simulink model "SimParking"  (R2017b)
settings: Solver=VariableStepAuto  StartTime=0.0  StopTime=1761  RelTol=1e-3
libraries: neural x1111
(part 3 of 60)

== system SimParking/BestNet- 10 delays -100 100 hidden neurons/Layer 2 ==
  "a{1} " : Inport  PortDimensions=100  SampleTime=1
      mask Display: e = 0.06;c1 = [120 230 180]/255;c2 = ([120 230 180]+0)/(256+128);c3 = ([120 230 180]+128)/(256+128);patch([0 1 1 0],[0 0 1 1],c1);patch([0 1 1 1-e 1-e 0+e],[0 0 1 1-e 0+e 0+e],c2);patch([0 0 1 1-e 0+e 0+e],[0 1 1 1-e 1-e 0+e],c3);plot([0 1 1 0 0],[0 0 1 1 0]);
  Delays 1 : Subsystem
      mask Display: e = 0.06;c1 = [120 150 230]/255;c2 = ([120 150 230]+0)/383;c3 = ([120 150 230]+128)/383;patch([0 1 1 0],[0 0 1 1],c1);patch([0 1 1 1-e 1-e 0+e],[0 0 1 1-e 0+e 0+e],c2);patch([0 0 1 1-e 0+e 0+e],[0 1 1 1-e 1-e 0+e],c3);plot([0 1 1 0 0],[0 0 1 1 0]);disp('0');
  "LW{2,1}" : Subsystem
      mask Display: e = 0.06;c1 = [120 150 230]/255;c2 = ([120 150 230]+0)/383;c3 = ([120 150 230]+128)/383;patch([0 1 1 0],[0 0 1 1],c1);patch([0 1 1 1-e 1-e 0+e],[0 0 1 1-e 0+e 0+e],c2);patch([0 0 1 1-e 0+e 0+e],[0 1 1 1-e 1-e 0+e],c3);plot([0 1 1 0 0],[0 0 1 1 0]);disp('W');
  "b{2}" : Constant  Value=[-1.5233467696368359067804476580931805074214935302734375;-1.4415804453285188113653703112504445016384124755859375;1.4687499329954964988331767017371021211147308349609375;1.378535301430398707367430688464082777500152587890625;1.4334155218379340812617783740279264748096466064453125;-1.3690887831616393999212277776678092777729034423828125;-1.304160375402110272347044883645139634609222412109375;1.29600772472264846868483800790272653102874755859375;1.2498985632110517496329293862800113856792449951171875;1.2638509294992459341955282070557586848735809326171875;1.208129855846170830346864022430963814258575439453125;1.1824187437823148183468902061576955020427703857421875;1.160993267964341324471888583502732217311859130859375;1.10675966022170069180674545350484549999237060546875;-1.105033867711343820161573603400029242038726806640625;1.032881951698968681085943899233825504779815673828125;-0.98852583000171645455367297472548671066761016845703125;-1.003489835974161525911085846018977463245391845703125;-0.94450071591520201597091954681673087179660797119140625;-0.96655837310848158328013823847868479788303375244140625;-0.8538722720434481772144863498397171497344970703125;0.8426292105943014032476412467076443135738372802734375;-0.8802935092119688054168591406778432428836822509765625;-0.81787353156131759046587603734224103391170501708984375;-0.7137736873323863306950443075038492679595947265625;-0.7368245035904037454344006619066931307315826416015625;-0.66775958311495842156801927558262832462787628173828125;-0.57961887312592608179073749852250330150127410888671875;0.67555184756865627182520483984262682497501373291015625;0.68969451052878183450189908398897387087345123291015625;0.61762410004044998590444492947426624596118927001953125;0.6022014857071804616595045445137657225131988525390625;-0.526192511812102026169668533839285373687744140625;0.51561667677955635991082772306981496512889862060546875;-0.414470085354920747544582582122529856860637664794921875;-0.43640562865662513303277592058293521404266357421875;-0.4769010705651643977631692905561067163944244384765625;0.30156500972384758796351889031939208507537841796875;0.380377257082855357861461698121274821460247039794921875;-0.256097557968687272733632198651321232318878173828125;0.25819514267073084834436258461209945380687713623046875;0.239800622449258538093630477305850945413112640380859375;0.238207291683244115620965430935029871761798858642578125;-0.2465816261413751597775245727461879141628742218017578125;0.2765787596096604961104503672686405479907989501953125;0.08005536680915757707932556286323233507573604583740234375;-0.1529351096854706659744493890684680081903934478759765625;0.11905624484543265995117877764641889370977878570556640625;0.09813681425791646872891504926883499138057231903076171875;-0.0679352414639936286189225711495964787900447845458984375;-0.06834830466920095715099847666351706720888614654541015625;-0.156043028201395816978447328438051044940948486328125;0.0237726502873336666132875194534790352918207645416259765625;-0.034534939705202348514401222701053484342992305755615234375;-0.042901038724158180315271238214336335659027099609375;0.1717782700492356540156180244593997485935688018798828125;0.1147508327533348360116605135772260837256908416748046875;-0.254165471349188598626511748079792596399784088134765625;0.2069296799639553097183153340665739960968494415283203125;-0.29569483453317657595249556834460236132144927978515625;0.388897541037930560836599624963128007948398590087890625;-0.373484441161281266463589645354659296572208404541015625;-0.363064211852830276416881361001287586987018585205078125;-0.40194412444326232947133803463657386600971221923828125;0.52257111750173967923416284975246526300907135009765625;-0.4052040280159545648785979210515506565570831298828125;0.4311907495262088385601373374811373651027679443359375;0.623613308142939803957460753736086189746856689453125;-0.485832292806824661557385525156860239803791046142578125;-0.66397809913526162350905224229791201651096343994140625;-0.672562449456481470377866571652702987194061279296875 ...(+1576 chars)]
      mask Display: e = 0.06;c1 = [120 150 230]/255;c2 = ([120 150 230]+0)/383;c3 = ([120 150 230]+128)/383;patch([0 1 1 0],[0 0 1 1],c1);patch([0 1 1 1-e 1-e 0+e],[0 0 1 1-e 0+e 0+e],c2);patch([0 0 1 1-e 0+e 0+e],[0 1 1 1-e 1-e 0+e],c3);plot([0 1 1 0 0],[0 0 1 1 0]);disp('b');
  netsum : Sum  Inputs=2  SaturateOnIntegerOverflow=on  InputSameDT=on  OutDataTypeStr=Inherit: Same as first input
      mask Display: e = 0.06;c1 = [120 150 230]/255;c2 = ([120 150 230]+0)/383;c3 = ([120 150 230]+128)/383;patch([0 1 1 0],[0 0 1 1],c1);patch([0 1 1 1-e 1-e 0+e],[0 0 1 1-e 0+e 0+e],c2);patch([0 0 1 1-e 0+e 0+e],[0 1 1 1-e 1-e 0+e],c3);plot([0 1 1 0 0],[0 0 1 1 0]);disp('+');
  tansig : neural/Transfer Functions/tansig
  "a{2}" : Outport  InitialOutput=[0;0;0;0;0;0;0;0;0;0;0;0;0;0;0;0;0;0;0;0;0;0;0;0;0;0;0;0;0;0;0;0;0;0;0;0;0;0;0;0;0;0;0;0;0;0;0;0;0;0;0;0;0;0;0;0;0;0;0;0;0;0;0;0;0;0;0;0;0;0;0;0;0;0;0;0;0;0;0;0;0;0;0;0;0;0;0;0;0;0;0;0;0;0;0;0;0;0;0;0]
      mask Display: e = 0.06;c1 = [120 230 180]/255;c2 = ([120 230 180]+0)/(256+128);c3 = ([120 230 180]+128)/(256+128);patch([0 1 1 0],[0 0 1 1],c1);patch([0 1 1 1-e 1-e 0+e],[0 0 1 1-e 0+e 0+e],c2);patch([0 0 1 1-e 0+e 0+e],[0 1 1 1-e 1-e 0+e],c3);plot([0 1 1 0 0],[0 0 1 1 0]);
  wires:
  "a{1} "/1 -> Delays 1/1("p{2}")
  Delays 1/1("pd{2,1}") -> "LW{2,1}"/1("ad{2,1}")
  "LW{2,1}"/1("lz{2,1}") -> netsum/1
  "b{2}"/1 -> netsum/2
  netsum/1 -> tansig/1
  tansig/1 -> "a{2}"/1

== system SimParking/BestNet- 10 delays -100 100 hidden neurons/Layer 3 ==
  "a{2} " : Inport  PortDimensions=100  SampleTime=1
      mask Display: e = 0.06;c1 = [120 230 180]/255;c2 = ([120 230 180]+0)/(256+128);c3 = ([120 230 180]+128)/(256+128);patch([0 1 1 0],[0 0 1 1],c1);patch([0 1 1 1-e 1-e 0+e],[0 0 1 1-e 0+e 0+e],c2);patch([0 0 1 1-e 0+e 0+e],[0 1 1 1-e 1-e 0+e],c3);plot([0 1 1 0 0],[0 0 1 1 0]);
  Delays 1 : Subsystem
      mask Display: e = 0.06;c1 = [120 150 230]/255;c2 = ([120 150 230]+0)/383;c3 = ([120 150 230]+128)/383;patch([0 1 1 0],[0 0 1 1],c1);patch([0 1 1 1-e 1-e 0+e],[0 0 1 1-e 0+e 0+e],c2);patch([0 0 1 1-e 0+e 0+e],[0 1 1 1-e 1-e 0+e],c3);plot([0 1 1 0 0],[0 0 1 1 0]);disp('0');
  "LW{3,2}" : Subsystem
      mask Display: e = 0.06;c1 = [120 150 230]/255;c2 = ([120 150 230]+0)/383;c3 = ([120 150 230]+128)/383;patch([0 1 1 0],[0 0 1 1],c1);patch([0 1 1 1-e 1-e 0+e],[0 0 1 1-e 0+e 0+e],c2);patch([0 0 1 1-e 0+e 0+e],[0 1 1 1-e 1-e 0+e],c3);plot([0 1 1 0 0],[0 0 1 1 0]);disp('W');
  "b{3}" : Constant  Value=[-0.264399040939169382991025258888839744031429290771484375;-0.2280200632373896307836247387967887334525585174560546875;0.1500776635383979928928255276332492940127849578857421875]
      mask Display: e = 0.06;c1 = [120 150 230]/255;c2 = ([120 150 230]+0)/383;c3 = ([120 150 230]+128)/383;patch([0 1 1 0],[0 0 1 1],c1);patch([0 1 1 1-e 1-e 0+e],[0 0 1 1-e 0+e 0+e],c2);patch([0 0 1 1-e 0+e 0+e],[0 1 1 1-e 1-e 0+e],c3);plot([0 1 1 0 0],[0 0 1 1 0]);disp('b');
  netsum : Sum  Inputs=2  SaturateOnIntegerOverflow=on  InputSameDT=on  OutDataTypeStr=Inherit: Same as first input
      mask Display: e = 0.06;c1 = [120 150 230]/255;c2 = ([120 150 230]+0)/383;c3 = ([120 150 230]+128)/383;patch([0 1 1 0],[0 0 1 1],c1);patch([0 1 1 1-e 1-e 0+e],[0 0 1 1-e 0+e 0+e],c2);patch([0 0 1 1-e 0+e 0+e],[0 1 1 1-e 1-e 0+e],c3);plot([0 1 1 0 0],[0 0 1 1 0]);disp('+');
  purelin : neural/Transfer Functions/purelin
  "a{3}" : Outport  InitialOutput=[0;0;0]
      mask Display: e = 0.06;c1 = [120 230 180]/255;c2 = ([120 230 180]+0)/(256+128);c3 = ([120 230 180]+128)/(256+128);patch([0 1 1 0],[0 0 1 1],c1);patch([0 1 1 1-e 1-e 0+e],[0 0 1 1-e 0+e 0+e],c2);patch([0 0 1 1-e 0+e 0+e],[0 1 1 1-e 1-e 0+e],c3);plot([0 1 1 0 0],[0 0 1 1 0]);
  wires:
  "a{2} "/1 -> Delays 1/1("p{3}")
  Delays 1/1("pd{3,2}") -> "LW{3,2}"/1("ad{3,2}")
  "LW{3,2}"/1("lz{3,2}") -> netsum/1
  "b{3}"/1 -> netsum/2
  netsum/1 -> purelin/1
  purelin/1 -> "a{3}"/1

== system SimParking/BestNet- 10 delays -100 100 hidden neurons/Process Input 1 ==
  x : Inport  PortDimensions=9  SampleTime=1
      mask Display: e = 0.06;c1 = [120 230 180]/255;c2 = ([120 230 180]+0)/(256+128);c3 = ([120 230 180]+128)/(256+128);patch([0 1 1 0],[0 0 1 1],c1);patch([0 1 1 1-e 1-e 0+e],[0 0 1 1-e 0+e 0+e],c2);patch([0 0 1 1-e 0+e 0+e],[0 1 1 1-e 1-e 0+e],c3);plot([0 1 1 0 0],[0 0 1 1 0]);
  mapminmax : neural/Processing Functions/mapminmax  xmin=[0;-0.00100000000000000002081668171172;-0.927000000000000046185277824407;-0.0367373000000000005105249556436;0;0;0;0;0]  xmax=[1;4.75300000000000011368683772162;0;1.1136800000000000032684965845;2.19799999999999995381472217559;1;1;1;1]  ymin=-1  ymax=1
  p : Outport  PortDimensions=9  SampleTime=1
      mask Display: e = 0.06;c1 = [120 230 180]/255;c2 = ([120 230 180]+0)/(256+128);c3 = ([120 230 180]+128)/(256+128);patch([0 1 1 0],[0 0 1 1],c1);patch([0 1 1 1-e 1-e 0+e],[0 0 1 1-e 0+e 0+e],c2);patch([0 0 1 1-e 0+e 0+e],[0 1 1 1-e 1-e 0+e],c3);plot([0 1 1 0 0],[0 0 1 1 0]);
  wires:
  x/1 -> mapminmax/1
  mapminmax/1 -> p/1

== system SimParking/BestNet- 10 delays -100 100 hidden neurons/Process Output 1 ==
  a : Inport  PortDimensions=3  SampleTime=1
      mask Display: e = 0.06;c1 = [120 230 180]/255;c2 = ([120 230 180]+0)/(256+128);c3 = ([120 230 180]+128)/(256+128);patch([0 1 1 0],[0 0 1 1],c1);patch([0 1 1 1-e 1-e 0+e],[0 0 1 1-e 0+e 0+e],c2);patch([0 0 1 1-e 0+e 0+e],[0 1 1 1-e 1-e 0+e],c3);plot([0 1 1 0 0],[0 0 1 1 0]);
  mapminmax_reverse : neural/Processing Functions/mapminmax_reverse  xmin=[-0.142810999999999993503863038313;-0.169776000000000010237144465464;0]  xmax=[0.231192000000000008608225243734;0.179999999999999993338661852249;1]  ymin=-1  ymax=1
  y : Outport  PortDimensions=3  SampleTime=1
      mask Display: e = 0.06;c1 = [120 230 180]/255;c2 = ([120 230 180]+0)/(256+128);c3 = ([120 230 180]+128)/(256+128);patch([0 1 1 0],[0 0 1 1],c1);patch([0 1 1 1-e 1-e 0+e],[0 0 1 1-e 0+e 0+e],c2);patch([0 0 1 1-e 0+e 0+e],[0 1 1 1-e 1-e 0+e],c3);plot([0 1 1 0 0],[0 0 1 1 0]);
  wires:
  a/1 -> mapminmax_reverse/1
  mapminmax_reverse/1 -> y/1

== system SimParking/BestNet- 10 delays -100 100 hidden neurons1/Layer 1 ==
  "p{1}" : Inport  PortDimensions=9  SampleTime=1
      mask Display: e = 0.06;c1 = [120 230 180]/255;c2 = ([120 230 180]+0)/(256+128);c3 = ([120 230 180]+128)/(256+128);patch([0 1 1 0],[0 0 1 1],c1);patch([0 1 1 1-e 1-e 0+e],[0 0 1 1-e 0+e 0+e],c2);patch([0 0 1 1-e 0+e 0+e],[0 1 1 1-e 1-e 0+e],c3);plot([0 1 1 0 0],[0 0 1 1 0]);
  Delays 1 : Subsystem
      mask Display: e = 0.06;c1 = [120 150 230]/255;c2 = ([120 150 230]+0)/383;c3 = ([120 150 230]+128)/383;patch([0 1 1 0],[0 0 1 1],c1);patch([0 1 1 1-e 1-e 0+e],[0 0 1 1-e 0+e 0+e],c2);patch([0 0 1 1-e 0+e 0+e],[0 1 1 1-e 1-e 0+e],c3);plot([0 1 1 0 0],[0 0 1 1 0]);disp('1-10');
  "IW{1,1}" : Subsystem
      mask Display: e = 0.06;c1 = [120 150 230]/255;c2 = ([120 150 230]+0)/383;c3 = ([120 150 230]+128)/383;patch([0 1 1 0],[0 0 1 1],c1);patch([0 1 1 1-e 1-e 0+e],[0 0 1 1-e 0+e 0+e],c2);patch([0 0 1 1-e 0+e 0+e],[0 1 1 1-e 1-e 0+e],c3);plot([0 1 1 0 0],[0 0 1 1 0]);disp('W');
  "b{1}" : Constant  Value=[-1.5245225286757662086500886289286427199840545654296875;1.6058316686755433888578181722550652921199798583984375;1.517403103952690290867622024961747229099273681640625;-1.386904812575269207997052944847382605075836181640625;-1.3545623995403683892391200060956180095672607421875;1.470857444827213367233298413339070975780487060546875;-1.2857387543680351971175923608825542032718658447265625;-1.359082929289666452632445725612342357635498046875;-1.3064762119514614635562566036242060363292694091796875;-1.22721098835727193687716862768866121768951416015625;1.2308531077143507470594840924604795873165130615234375;1.336790839668508201754093533963896334171295166015625;1.11248789445838536238397864508442580699920654296875;1.161779163995248609353438951075077056884765625;-1.11085814127999693567971917218528687953948974609375;-1.16588845394895290752401706413365900516510009765625;0.978431286318926396461392869241535663604736328125;-1.0267597507064201156623539645806886255741119384765625;-1.0466534182444442446779930833145044744014739990234375;1.05098808141578725638964897370897233486175537109375;0.93621859385301731126816093819797970354557037353515625;-1.000511208787383310436780448071658611297607421875;-0.90766483038739564914720858723740093410015106201171875;-0.84546048837210940885000809430493973195552825927734375;0.84876630264789287849680476938374340534210205078125;-0.80185690636105755313423060215427540242671966552734375;-0.5148210028828319462235185710596852004528045654296875;-0.65524102483332169466478944741538725793361663818359375;0.715828663178128099531249972642399370670318603515625;0.547477588095126588285666002775542438030242919921875;0.6337090972519561216103056722204200923442840576171875;0.61282296794795898531305056167184375226497650146484375;-0.62963945517072217317178228768170811235904693603515625;-0.5600633886452470733274822123348712921142578125;-0.5142547132588661806806840104400180280208587646484375;0.36622414618450871426347248416277579963207244873046875;0.435171860018647882473175059203640557825565338134765625;-0.3973775967826436161800529589527286589145660400390625;-0.412985049052973895999940623369184322655200958251953125;-0.456498738819200500227424299737322144210338592529296875;-0.368563532068655719253769120768993161618709564208984375;-0.1451264394857011696959858682021149434149265289306640625;0.2374280696468461793191551123527460731565952301025390625;0.169516230719349125788397714131860993802547454833984375;-0.01207776799942027710910164017832357785664498805999755859375;0.07982326989852468746011737721346435137093067169189453125;0.18978690166193568078512043939554132521152496337890625;0.1312090183858221903445695488699129782617092132568359375;-0.13599776027038201764440827901125885546207427978515625;0.0259802672083776220457451699985540471971035003662109375;0.09588393978311908483203040987064014188945293426513671875;-0.000439077264281844520908693052518856347887776792049407958984375;0.10623277174090879626522365697383065707981586456298828125;-0.1382214176826130069830611546422005631029605865478515625;0.128992117787592286415332409887923859059810638427734375;-0.0820858742952841613504944007218000479042530059814453125;-0.1798165459899483398231723185745067894458770751953125;-0.386315691932279381415327179638552479445934295654296875;0.18505331061093144295881529615144245326519012451171875;-0.276070952220042686864331926699378527700901031494140625;0.1470903025261399432732645209398469887673854827880859375;0.355437619732055509746970756168593652546405792236328125;-0.33831043495201262860661017839447595179080963134765625;-0.507272391830840607696018196293152868747711181640625;0.459441289358410720478076427752966992557048797607421875;0.424515668838529147688376497171702794730663299560546875;0.63498576332306655434223330303211696445941925048828125;0.487893153924136402377342847103136591613292694091796875;0.69410429992965394507820064973202534019947052001953125;0.751872227891053679371680118492804467678070068359375;-0.82872934292105782105863909237086772918701171875 ...(+1580 chars)]
      mask Display: e = 0.06;c1 = [120 150 230]/255;c2 = ([120 150 230]+0)/383;c3 = ([120 150 230]+128)/383;patch([0 1 1 0],[0 0 1 1],c1);patch([0 1 1 1-e 1-e 0+e],[0 0 1 1-e 0+e 0+e],c2);patch([0 0 1 1-e 0+e 0+e],[0 1 1 1-e 1-e 0+e],c3);plot([0 1 1 0 0],[0 0 1 1 0]);disp('b');
  netsum : Sum  Inputs=2  SaturateOnIntegerOverflow=on  InputSameDT=on  OutDataTypeStr=Inherit: Same as first input
      mask Display: e = 0.06;c1 = [120 150 230]/255;c2 = ([120 150 230]+0)/383;c3 = ([120 150 230]+128)/383;patch([0 1 1 0],[0 0 1 1],c1);patch([0 1 1 1-e 1-e 0+e],[0 0 1 1-e 0+e 0+e],c2);patch([0 0 1 1-e 0+e 0+e],[0 1 1 1-e 1-e 0+e],c3);plot([0 1 1 0 0],[0 0 1 1 0]);disp('+');
  tansig : neural/Transfer Functions/tansig
  "a{1}" : Outport  InitialOutput=[0;0;0;0;0;0;0;0;0;0;0;0;0;0;0;0;0;0;0;0;0;0;0;0;0;0;0;0;0;0;0;0;0;0;0;0;0;0;0;0;0;0;0;0;0;0;0;0;0;0;0;0;0;0;0;0;0;0;0;0;0;0;0;0;0;0;0;0;0;0;0;0;0;0;0;0;0;0;0;0;0;0;0;0;0;0;0;0;0;0;0;0;0;0;0;0;0;0;0;0]
      mask Display: e = 0.06;c1 = [120 230 180]/255;c2 = ([120 230 180]+0)/(256+128);c3 = ([120 230 180]+128)/(256+128);patch([0 1 1 0],[0 0 1 1],c1);patch([0 1 1 1-e 1-e 0+e],[0 0 1 1-e 0+e 0+e],c2);patch([0 0 1 1-e 0+e 0+e],[0 1 1 1-e 1-e 0+e],c3);plot([0 1 1 0 0],[0 0 1 1 0]);
  wires:
  "p{1}"/1 -> Delays 1/1("p{1}")
  Delays 1/1("pd{1,1}") -> "IW{1,1}"/1("pd{1,1}")
  "IW{1,1}"/1("iz{1,1}") -> netsum/1
  "b{1}"/1 -> netsum/2
  netsum/1 -> tansig/1
  tansig/1 -> "a{1}"/1

== system SimParking/BestNet- 10 delays -100 100 hidden neurons1/Layer 2 ==
  "a{1} " : Inport  PortDimensions=100  SampleTime=1
      mask Display: e = 0.06;c1 = [120 230 180]/255;c2 = ([120 230 180]+0)/(256+128);c3 = ([120 230 180]+128)/(256+128);patch([0 1 1 0],[0 0 1 1],c1);patch([0 1 1 1-e 1-e 0+e],[0 0 1 1-e 0+e 0+e],c2);patch([0 0 1 1-e 0+e 0+e],[0 1 1 1-e 1-e 0+e],c3);plot([0 1 1 0 0],[0 0 1 1 0]);
  Delays 1 : Subsystem
      mask Display: e = 0.06;c1 = [120 150 230]/255;c2 = ([120 150 230]+0)/383;c3 = ([120 150 230]+128)/383;patch([0 1 1 0],[0 0 1 1],c1);patch([0 1 1 1-e 1-e 0+e],[0 0 1 1-e 0+e 0+e],c2);patch([0 0 1 1-e 0+e 0+e],[0 1 1 1-e 1-e 0+e],c3);plot([0 1 1 0 0],[0 0 1 1 0]);disp('0');
  "LW{2,1}" : Subsystem
      mask Display: e = 0.06;c1 = [120 150 230]/255;c2 = ([120 150 230]+0)/383;c3 = ([120 150 230]+128)/383;patch([0 1 1 0],[0 0 1 1],c1);patch([0 1 1 1-e 1-e 0+e],[0 0 1 1-e 0+e 0+e],c2);patch([0 0 1 1-e 0+e 0+e],[0 1 1 1-e 1-e 0+e],c3);plot([0 1 1 0 0],[0 0 1 1 0]);disp('W');
  "b{2}" : Constant  Value=[-1.5233467696368359067804476580931805074214935302734375;-1.4415804453285188113653703112504445016384124755859375;1.4687499329954964988331767017371021211147308349609375;1.378535301430398707367430688464082777500152587890625;1.4334155218379340812617783740279264748096466064453125;-1.3690887831616393999212277776678092777729034423828125;-1.304160375402110272347044883645139634609222412109375;1.29600772472264846868483800790272653102874755859375;1.2498985632110517496329293862800113856792449951171875;1.2638509294992459341955282070557586848735809326171875;1.208129855846170830346864022430963814258575439453125;1.1824187437823148183468902061576955020427703857421875;1.160993267964341324471888583502732217311859130859375;1.10675966022170069180674545350484549999237060546875;-1.105033867711343820161573603400029242038726806640625;1.032881951698968681085943899233825504779815673828125;-0.98852583000171645455367297472548671066761016845703125;-1.003489835974161525911085846018977463245391845703125;-0.94450071591520201597091954681673087179660797119140625;-0.96655837310848158328013823847868479788303375244140625;-0.8538722720434481772144863498397171497344970703125;0.8426292105943014032476412467076443135738372802734375;-0.8802935092119688054168591406778432428836822509765625;-0.81787353156131759046587603734224103391170501708984375;-0.7137736873323863306950443075038492679595947265625;-0.7368245035904037454344006619066931307315826416015625;-0.66775958311495842156801927558262832462787628173828125;-0.57961887312592608179073749852250330150127410888671875;0.67555184756865627182520483984262682497501373291015625;0.68969451052878183450189908398897387087345123291015625;0.61762410004044998590444492947426624596118927001953125;0.6022014857071804616595045445137657225131988525390625;-0.526192511812102026169668533839285373687744140625;0.51561667677955635991082772306981496512889862060546875;-0.414470085354920747544582582122529856860637664794921875;-0.43640562865662513303277592058293521404266357421875;-0.4769010705651643977631692905561067163944244384765625;0.30156500972384758796351889031939208507537841796875;0.380377257082855357861461698121274821460247039794921875;-0.256097557968687272733632198651321232318878173828125;0.25819514267073084834436258461209945380687713623046875;0.239800622449258538093630477305850945413112640380859375;0.238207291683244115620965430935029871761798858642578125;-0.2465816261413751597775245727461879141628742218017578125;0.2765787596096604961104503672686405479907989501953125;0.08005536680915757707932556286323233507573604583740234375;-0.1529351096854706659744493890684680081903934478759765625;0.11905624484543265995117877764641889370977878570556640625;0.09813681425791646872891504926883499138057231903076171875;-0.0679352414639936286189225711495964787900447845458984375;-0.06834830466920095715099847666351706720888614654541015625;-0.156043028201395816978447328438051044940948486328125;0.0237726502873336666132875194534790352918207645416259765625;-0.034534939705202348514401222701053484342992305755615234375;-0.042901038724158180315271238214336335659027099609375;0.1717782700492356540156180244593997485935688018798828125;0.1147508327533348360116605135772260837256908416748046875;-0.254165471349188598626511748079792596399784088134765625;0.2069296799639553097183153340665739960968494415283203125;-0.29569483453317657595249556834460236132144927978515625;0.388897541037930560836599624963128007948398590087890625;-0.373484441161281266463589645354659296572208404541015625;-0.363064211852830276416881361001287586987018585205078125;-0.40194412444326232947133803463657386600971221923828125;0.52257111750173967923416284975246526300907135009765625;-0.4052040280159545648785979210515506565570831298828125;0.4311907495262088385601373374811373651027679443359375;0.623613308142939803957460753736086189746856689453125;-0.485832292806824661557385525156860239803791046142578125;-0.66397809913526162350905224229791201651096343994140625;-0.672562449456481470377866571652702987194061279296875 ...(+1576 chars)]
      mask Display: e = 0.06;c1 = [120 150 230]/255;c2 = ([120 150 230]+0)/383;c3 = ([120 150 230]+128)/383;patch([0 1 1 0],[0 0 1 1],c1);patch([0 1 1 1-e 1-e 0+e],[0 0 1 1-e 0+e 0+e],c2);patch([0 0 1 1-e 0+e 0+e],[0 1 1 1-e 1-e 0+e],c3);plot([0 1 1 0 0],[0 0 1 1 0]);disp('b');
  netsum : Sum  Inputs=2  SaturateOnIntegerOverflow=on  InputSameDT=on  OutDataTypeStr=Inherit: Same as first input
      mask Display: e = 0.06;c1 = [120 150 230]/255;c2 = ([120 150 230]+0)/383;c3 = ([120 150 230]+128)/383;patch([0 1 1 0],[0 0 1 1],c1);patch([0 1 1 1-e 1-e 0+e],[0 0 1 1-e 0+e 0+e],c2);patch([0 0 1 1-e 0+e 0+e],[0 1 1 1-e 1-e 0+e],c3);plot([0 1 1 0 0],[0 0 1 1 0]);disp('+');
  tansig : neural/Transfer Functions/tansig
  "a{2}" : Outport  InitialOutput=[0;0;0;0;0;0;0;0;0;0;0;0;0;0;0;0;0;0;0;0;0;0;0;0;0;0;0;0;0;0;0;0;0;0;0;0;0;0;0;0;0;0;0;0;0;0;0;0;0;0;0;0;0;0;0;0;0;0;0;0;0;0;0;0;0;0;0;0;0;0;0;0;0;0;0;0;0;0;0;0;0;0;0;0;0;0;0;0;0;0;0;0;0;0;0;0;0;0;0;0]
      mask Display: e = 0.06;c1 = [120 230 180]/255;c2 = ([120 230 180]+0)/(256+128);c3 = ([120 230 180]+128)/(256+128);patch([0 1 1 0],[0 0 1 1],c1);patch([0 1 1 1-e 1-e 0+e],[0 0 1 1-e 0+e 0+e],c2);patch([0 0 1 1-e 0+e 0+e],[0 1 1 1-e 1-e 0+e],c3);plot([0 1 1 0 0],[0 0 1 1 0]);
  wires:
  "a{1} "/1 -> Delays 1/1("p{2}")
  Delays 1/1("pd{2,1}") -> "LW{2,1}"/1("ad{2,1}")
  "LW{2,1}"/1("lz{2,1}") -> netsum/1
  "b{2}"/1 -> netsum/2
  netsum/1 -> tansig/1
  tansig/1 -> "a{2}"/1

== system SimParking/BestNet- 10 delays -100 100 hidden neurons1/Layer 3 ==
  "a{2} " : Inport  PortDimensions=100  SampleTime=1
      mask Display: e = 0.06;c1 = [120 230 180]/255;c2 = ([120 230 180]+0)/(256+128);c3 = ([120 230 180]+128)/(256+128);patch([0 1 1 0],[0 0 1 1],c1);patch([0 1 1 1-e 1-e 0+e],[0 0 1 1-e 0+e 0+e],c2);patch([0 0 1 1-e 0+e 0+e],[0 1 1 1-e 1-e 0+e],c3);plot([0 1 1 0 0],[0 0 1 1 0]);
  Delays 1 : Subsystem
      mask Display: e = 0.06;c1 = [120 150 230]/255;c2 = ([120 150 230]+0)/383;c3 = ([120 150 230]+128)/383;patch([0 1 1 0],[0 0 1 1],c1);patch([0 1 1 1-e 1-e 0+e],[0 0 1 1-e 0+e 0+e],c2);patch([0 0 1 1-e 0+e 0+e],[0 1 1 1-e 1-e 0+e],c3);plot([0 1 1 0 0],[0 0 1 1 0]);disp('0');
  "LW{3,2}" : Subsystem
      mask Display: e = 0.06;c1 = [120 150 230]/255;c2 = ([120 150 230]+0)/383;c3 = ([120 150 230]+128)/383;patch([0 1 1 0],[0 0 1 1],c1);patch([0 1 1 1-e 1-e 0+e],[0 0 1 1-e 0+e 0+e],c2);patch([0 0 1 1-e 0+e 0+e],[0 1 1 1-e 1-e 0+e],c3);plot([0 1 1 0 0],[0 0 1 1 0]);disp('W');
  "b{3}" : Constant  Value=[-0.264399040939169382991025258888839744031429290771484375;-0.2280200632373896307836247387967887334525585174560546875;0.1500776635383979928928255276332492940127849578857421875]
      mask Display: e = 0.06;c1 = [120 150 230]/255;c2 = ([120 150 230]+0)/383;c3 = ([120 150 230]+128)/383;patch([0 1 1 0],[0 0 1 1],c1);patch([0 1 1 1-e 1-e 0+e],[0 0 1 1-e 0+e 0+e],c2);patch([0 0 1 1-e 0+e 0+e],[0 1 1 1-e 1-e 0+e],c3);plot([0 1 1 0 0],[0 0 1 1 0]);disp('b');
  netsum : Sum  Inputs=2  SaturateOnIntegerOverflow=on  InputSameDT=on  OutDataTypeStr=Inherit: Same as first input
      mask Display: e = 0.06;c1 = [120 150 230]/255;c2 = ([120 150 230]+0)/383;c3 = ([120 150 230]+128)/383;patch([0 1 1 0],[0 0 1 1],c1);patch([0 1 1 1-e 1-e 0+e],[0 0 1 1-e 0+e 0+e],c2);patch([0 0 1 1-e 0+e 0+e],[0 1 1 1-e 1-e 0+e],c3);plot([0 1 1 0 0],[0 0 1 1 0]);disp('+');
  purelin : neural/Transfer Functions/purelin
  "a{3}" : Outport  InitialOutput=[0;0;0]
      mask Display: e = 0.06;c1 = [120 230 180]/255;c2 = ([120 230 180]+0)/(256+128);c3 = ([120 230 180]+128)/(256+128);patch([0 1 1 0],[0 0 1 1],c1);patch([0 1 1 1-e 1-e 0+e],[0 0 1 1-e 0+e 0+e],c2);patch([0 0 1 1-e 0+e 0+e],[0 1 1 1-e 1-e 0+e],c3);plot([0 1 1 0 0],[0 0 1 1 0]);
  wires:
  "a{2} "/1 -> Delays 1/1("p{3}")
  Delays 1/1("pd{3,2}") -> "LW{3,2}"/1("ad{3,2}")
  "LW{3,2}"/1("lz{3,2}") -> netsum/1
  "b{3}"/1 -> netsum/2
  netsum/1 -> purelin/1
  purelin/1 -> "a{3}"/1

== system SimParking/BestNet- 10 delays -100 100 hidden neurons1/Process Input 1 ==
  x : Inport  PortDimensions=9  SampleTime=1
      mask Display: e = 0.06;c1 = [120 230 180]/255;c2 = ([120 230 180]+0)/(256+128);c3 = ([120 230 180]+128)/(256+128);patch([0 1 1 0],[0 0 1 1],c1);patch([0 1 1 1-e 1-e 0+e],[0 0 1 1-e 0+e 0+e],c2);patch([0 0 1 1-e 0+e 0+e],[0 1 1 1-e 1-e 0+e],c3);plot([0 1 1 0 0],[0 0 1 1 0]);
  mapminmax : neural/Processing Functions/mapminmax  xmin=[0;-0.00100000000000000002081668171172;-0.927000000000000046185277824407;-0.0367373000000000005105249556436;0;0;0;0;0]  xmax=[1;4.75300000000000011368683772162;0;1.1136800000000000032684965845;2.19799999999999995381472217559;1;1;1;1]  ymin=-1  ymax=1
  p : Outport  PortDimensions=9  SampleTime=1
      mask Display: e = 0.06;c1 = [120 230 180]/255;c2 = ([120 230 180]+0)/(256+128);c3 = ([120 230 180]+128)/(256+128);patch([0 1 1 0],[0 0 1 1],c1);patch([0 1 1 1-e 1-e 0+e],[0 0 1 1-e 0+e 0+e],c2);patch([0 0 1 1-e 0+e 0+e],[0 1 1 1-e 1-e 0+e],c3);plot([0 1 1 0 0],[0 0 1 1 0]);
  wires:
  x/1 -> mapminmax/1
  mapminmax/1 -> p/1

== system SimParking/BestNet- 10 delays -100 100 hidden neurons1/Process Output 1 ==
  a : Inport  PortDimensions=3  SampleTime=1
      mask Display: e = 0.06;c1 = [120 230 180]/255;c2 = ([120 230 180]+0)/(256+128);c3 = ([120 230 180]+128)/(256+128);patch([0 1 1 0],[0 0 1 1],c1);patch([0 1 1 1-e 1-e 0+e],[0 0 1 1-e 0+e 0+e],c2);patch([0 0 1 1-e 0+e 0+e],[0 1 1 1-e 1-e 0+e],c3);plot([0 1 1 0 0],[0 0 1 1 0]);
  mapminmax_reverse : neural/Processing Functions/mapminmax_reverse  xmin=[-0.142810999999999993503863038313;-0.169776000000000010237144465464;0]  xmax=[0.231192000000000008608225243734;0.179999999999999993338661852249;1]  ymin=-1  ymax=1
  y : Outport  PortDimensions=3  SampleTime=1
      mask Display: e = 0.06;c1 = [120 230 180]/255;c2 = ([120 230 180]+0)/(256+128);c3 = ([120 230 180]+128)/(256+128);patch([0 1 1 0],[0 0 1 1],c1);patch([0 1 1 1-e 1-e 0+e],[0 0 1 1-e 0+e 0+e],c2);patch([0 0 1 1-e 0+e 0+e],[0 1 1 1-e 1-e 0+e],c3);plot([0 1 1 0 0],[0 0 1 1 0]);
  wires:
  a/1 -> mapminmax_reverse/1
  mapminmax_reverse/1 -> y/1

== system SimParking/NARX Neural Network/Layer 1 ==
  "p{1}" : Inport  PortDimensions=9  SampleTime=1
      mask Display: e = 0.06;c1 = [120 230 180]/255;c2 = ([120 230 180]+0)/(256+128);c3 = ([120 230 180]+128)/(256+128);patch([0 1 1 0],[0 0 1 1],c1);patch([0 1 1 1-e 1-e 0+e],[0 0 1 1-e 0+e 0+e],c2);patch([0 0 1 1-e 0+e 0+e],[0 1 1 1-e 1-e 0+e],c3);plot([0 1 1 0 0],[0 0 1 1 0]);
  "p{2}" : Inport  Port=2  PortDimensions=3  SampleTime=1
      mask Display: e = 0.06;c1 = [120 230 180]/255;c2 = ([120 230 180]+0)/(256+128);c3 = ([120 230 180]+128)/(256+128);patch([0 1 1 0],[0 0 1 1],c1);patch([0 1 1 1-e 1-e 0+e],[0 0 1 1-e 0+e 0+e],c2);patch([0 0 1 1-e 0+e 0+e],[0 1 1 1-e 1-e 0+e],c3);plot([0 1 1 0 0],[0 0 1 1 0]);
  Delays 1 : Subsystem
      mask Display: e = 0.06;c1 = [120 150 230]/255;c2 = ([120 150 230]+0)/383;c3 = ([120 150 230]+128)/383;patch([0 1 1 0],[0 0 1 1],c1);patch([0 1 1 1-e 1-e 0+e],[0 0 1 1-e 0+e 0+e],c2);patch([0 0 1 1-e 0+e 0+e],[0 1 1 1-e 1-e 0+e],c3);plot([0 1 1 0 0],[0 0 1 1 0]);disp('0');
  Delays 2 : Subsystem
      mask Display: e = 0.06;c1 = [120 150 230]/255;c2 = ([120 150 230]+0)/383;c3 = ([120 150 230]+128)/383;patch([0 1 1 0],[0 0 1 1],c1);patch([0 1 1 1-e 1-e 0+e],[0 0 1 1-e 0+e 0+e],c2);patch([0 0 1 1-e 0+e 0+e],[0 1 1 1-e 1-e 0+e],c3);plot([0 1 1 0 0],[0 0 1 1 0]);disp('1-50');
  "IW{1,1}" : Subsystem
      mask Display: e = 0.06;c1 = [120 150 230]/255;c2 = ([120 150 230]+0)/383;c3 = ([120 150 230]+128)/383;patch([0 1 1 0],[0 0 1 1],c1);patch([0 1 1 1-e 1-e 0+e],[0 0 1 1-e 0+e 0+e],c2);patch([0 0 1 1-e 0+e 0+e],[0 1 1 1-e 1-e 0+e],c3);plot([0 1 1 0 0],[0 0 1 1 0]);disp('W');
  "IW{1,2}" : Subsystem
      mask Display: e = 0.06;c1 = [120 150 230]/255;c2 = ([120 150 230]+0)/383;c3 = ([120 150 230]+128)/383;patch([0 1 1 0],[0 0 1 1],c1);patch([0 1 1 1-e 1-e 0+e],[0 0 1 1-e 0+e 0+e],c2);patch([0 0 1 1-e 0+e 0+e],[0 1 1 1-e 1-e 0+e],c3);plot([0 1 1 0 0],[0 0 1 1 0]);disp('W');
  "b{1}" : Constant  Value=[1.5969046224965197655620841032941825687885284423828125;-1.7912063546347847253770169118070043623447418212890625;-1.5388561055142222500080606550909578800201416015625;-1.41012773428703308553622264298610389232635498046875;1.2516979687990243963469083610107190907001495361328125;1.312373960278177431604262892506085336208343505859375;-0.983412682544885452529115354991517961025238037109375;-0.80986485866175794701149470711243338882923126220703125;-1.2029339295368204343361639985232613980770111083984375;-1.1670293037500563126940278380061499774456024169921875;0.77190111004026917829179410546203143894672393798828125;1.1170796386146815137863086420111358165740966796875;-0.9027681082827798686452069887309335172176361083984375;-0.84404484348430319773370911207166500389575958251953125;-0.8398823402892088285653926504892297089099884033203125;-0.96096732227412717808334718938567675650119781494140625;-0.80888228264187767013737584420596249401569366455078125;-0.8839470212697604356577585349441505968570709228515625;-0.5199915645703345745687329326756298542022705078125;-0.55491138067679290912792566814459860324859619140625;-0.2355995763063769843359551714456756599247455596923828125;0.1786679101826449678203090343231451697647571563720703125;0.06669160357916993631111068907557637430727481842041015625;0.33760169595970268563434046882321126759052276611328125;0.0640722658994543337040994401831994764506816864013671875;0.11033329275907544086976486141793429851531982421875;-0.02694162162876238830744313190734828822314739227294921875;0.07867268608938750296122321969960466958582401275634765625;-0.21652187256782118307540940804756246507167816162109375;-0.400963337846383105489422860046033747494220733642578125;0.49121250537639571387416026482242159545421600341796875;0.32538744056889534750354187053744681179523468017578125;-0.322036889699439277112702484373585321009159088134765625;-0.330652169761622649613030944237834773957729339599609375;-0.5574307196981103107447097499971278011798858642578125;-0.71726062559180137068182148141204379498958587646484375;-0.6226792083465870764058536224183626472949981689453125;0.5401443721909060524666301716933958232402801513671875;0.961042698197273725924105747253634035587310791015625;-0.8437616737450841508660914769279770553112030029296875;-0.969942042047644559232821848127059638500213623046875;-1.1821375776420401937372162137762643396854400634765625;1.27500930001485901499336250708438456058502197265625;1.1078610972992406491499650655896402895450592041015625;1.388994440773000604849585215561091899871826171875;-1.17813873765464283138726386823691427707672119140625;-1.4324081713273975058342557531432248651981353759765625;1.2708769176018248625581463784328661859035491943359375;-1.432438684290766151008256201748736202716827392578125;-1.6454473484770202329485755399218760430812835693359375]
      mask Display: e = 0.06;c1 = [120 150 230]/255;c2 = ([120 150 230]+0)/383;c3 = ([120 150 230]+128)/383;patch([0 1 1 0],[0 0 1 1],c1);patch([0 1 1 1-e 1-e 0+e],[0 0 1 1-e 0+e 0+e],c2);patch([0 0 1 1-e 0+e 0+e],[0 1 1 1-e 1-e 0+e],c3);plot([0 1 1 0 0],[0 0 1 1 0]);disp('b');
  netsum : Sum  Inputs=3  SaturateOnIntegerOverflow=on  InputSameDT=on  OutDataTypeStr=Inherit: Same as first input
      mask Display: e = 0.06;c1 = [120 150 230]/255;c2 = ([120 150 230]+0)/383;c3 = ([120 150 230]+128)/383;patch([0 1 1 0],[0 0 1 1],c1);patch([0 1 1 1-e 1-e 0+e],[0 0 1 1-e 0+e 0+e],c2);patch([0 0 1 1-e 0+e 0+e],[0 1 1 1-e 1-e 0+e],c3);plot([0 1 1 0 0],[0 0 1 1 0]);disp('+');
  tansig : neural/Transfer Functions/tansig
  "a{1}" : Outport  InitialOutput=[0;0;0;0;0;0;0;0;0;0;0;0;0;0;0;0;0;0;0;0;0;0;0;0;0;0;0;0;0;0;0;0;0;0;0;0;0;0;0;0;0;0;0;0;0;0;0;0;0;0]
      mask Display: e = 0.06;c1 = [120 230 180]/255;c2 = ([120 230 180]+0)/(256+128);c3 = ([120 230 180]+128)/(256+128);patch([0 1 1 0],[0 0 1 1],c1);patch([0 1 1 1-e 1-e 0+e],[0 0 1 1-e 0+e 0+e],c2);patch([0 0 1 1-e 0+e 0+e],[0 1 1 1-e 1-e 0+e],c3);plot([0 1 1 0 0],[0 0 1 1 0]);
  wires:
  "p{1}"/1 -> Delays 1/1("p{1}")
  Delays 1/1("pd{1,1}") -> "IW{1,1}"/1("pd{1,1}")
  "IW{1,1}"/1("iz{1,1}") -> netsum/1
  "p{2}"/1 -> Delays 2/1("p{1}")
  Delays 2/1("pd{1,2}") -> "IW{1,2}"/1("pd{1,2}")
  "IW{1,2}"/1("iz{1,2}") -> netsum/2
  "b{1}"/1 -> netsum/3
  netsum/1 -> tansig/1
  tansig/1 -> "a{1}"/1

== system SimParking/NARX Neural Network/Layer 2 ==
  "a{1} " : Inport  PortDimensions=50  SampleTime=1
      mask Display: e = 0.06;c1 = [120 230 180]/255;c2 = ([120 230 180]+0)/(256+128);c3 = ([120 230 180]+128)/(256+128);patch([0 1 1 0],[0 0 1 1],c1);patch([0 1 1 1-e 1-e 0+e],[0 0 1 1-e 0+e 0+e],c2);patch([0 0 1 1-e 0+e 0+e],[0 1 1 1-e 1-e 0+e],c3);plot([0 1 1 0 0],[0 0 1 1 0]);
  Delays 1 : Subsystem
      mask Display: e = 0.06;c1 = [120 150 230]/255;c2 = ([120 150 230]+0)/383;c3 = ([120 150 230]+128)/383;patch([0 1 1 0],[0 0 1 1],c1);patch([0 1 1 1-e 1-e 0+e],[0 0 1 1-e 0+e 0+e],c2);patch([0 0 1 1-e 0+e 0+e],[0 1 1 1-e 1-e 0+e],c3);plot([0 1 1 0 0],[0 0 1 1 0]);disp('0');
  "LW{2,1}" : Subsystem
      mask Display: e = 0.06;c1 = [120 150 230]/255;c2 = ([120 150 230]+0)/383;c3 = ([120 150 230]+128)/383;patch([0 1 1 0],[0 0 1 1],c1);patch([0 1 1 1-e 1-e 0+e],[0 0 1 1-e 0+e 0+e],c2);patch([0 0 1 1-e 0+e 0+e],[0 1 1 1-e 1-e 0+e],c3);plot([0 1 1 0 0],[0 0 1 1 0]);disp('W');
  "b{2}" : Constant  Value=[-1.6363503944643655874102705638506449759006500244140625;1.5360624516232579406249669773387722671031951904296875;1.11059861375738133659751838422380387783050537109375;-1.4392767505035759523224214717629365622997283935546875;1.4409351708761064525532447078148834407329559326171875;1.2175788630693633596280278652557171881198883056640625;1.3668542290579706044439944889745675027370452880859375;1.1700487481810857293140770707395859062671661376953125;-1.0419923047372190438863981398753821849822998046875;-1.0772920997316310920410842300043441355228424072265625;-0.92156744841401394552349302102811634540557861328125;0.65366594608739536642616485551116056740283966064453125;-0.78547397996821344268170150826335884630680084228515625;0.76072508917062686695231832345598377287387847900390625;-0.83257098268853757527807601945823989808559417724609375;0.66901667747235460392829509146395139396190643310546875;-0.63078423359023638727904881307040341198444366455078125;0.5420393016152809106955601237132214009761810302734375;-0.07946598732770930595403768847972969524562358856201171875;0.5423909762271801326960485312156379222869873046875;0.326606925114646007290986062798765487968921661376953125;0.3844185924897869366390068535110913217067718505859375;0.09491866885693635291776359963478171266615390777587890625;-0.25636261672081694928948536471580155193805694580078125;-0.2391039559703824479708345052131335251033306121826171875;-0.2132489161148002632106823739377432502806186676025390625;-0.00989623831989397927111351549456230713985860347747802734375;0.04987521390037075175172276431112550199031829833984375;0.5208785239988593662729954303358681499958038330078125;-0.395253894023191720830112672047107480466365814208984375;0.55574780083618957604585375520400702953338623046875;-0.50573626925899295425637092193937860429286956787109375;0.455131790521080048517177374378661625087261199951171875;0.6638857060691372158345302523230202496051788330078125;-0.82216853371897880009555592550896108150482177734375;0.757501367695529115309227563557215034961700439453125;0.79826921152868368647403940485673956573009490966796875;0.944106963196695847528872036491520702838897705078125;-0.963980899963555071252585548791103065013885498046875;1.0821648848898528516571104773902334272861480712890625;1.2086938644194600289694108141702599823474884033203125;1.0900749758012313606059251469559967517852783203125;1.15776420786700118270573511836118996143341064453125;1.19705558814239143572422108263708651065826416015625;1.283645721010774565229439758695662021636962890625;1.3018254109051115019468625177978537976741790771484375;-1.3466105406046164905120576804620213806629180908203125;1.6242884670598189966739255396532826125621795654296875;-1.5925514841884684802408855830435641109943389892578125;-1.5757390977362100148440049451892264187335968017578125]
      mask Display: e = 0.06;c1 = [120 150 230]/255;c2 = ([120 150 230]+0)/383;c3 = ([120 150 230]+128)/383;patch([0 1 1 0],[0 0 1 1],c1);patch([0 1 1 1-e 1-e 0+e],[0 0 1 1-e 0+e 0+e],c2);patch([0 0 1 1-e 0+e 0+e],[0 1 1 1-e 1-e 0+e],c3);plot([0 1 1 0 0],[0 0 1 1 0]);disp('b');
  netsum : Sum  Inputs=2  SaturateOnIntegerOverflow=on  InputSameDT=on  OutDataTypeStr=Inherit: Same as first input
      mask Display: e = 0.06;c1 = [120 150 230]/255;c2 = ([120 150 230]+0)/383;c3 = ([120 150 230]+128)/383;patch([0 1 1 0],[0 0 1 1],c1);patch([0 1 1 1-e 1-e 0+e],[0 0 1 1-e 0+e 0+e],c2);patch([0 0 1 1-e 0+e 0+e],[0 1 1 1-e 1-e 0+e],c3);plot([0 1 1 0 0],[0 0 1 1 0]);disp('+');
  tansig : neural/Transfer Functions/tansig
  "a{2}" : Outport  InitialOutput=[0;0;0;0;0;0;0;0;0;0;0;0;0;0;0;0;0;0;0;0;0;0;0;0;0;0;0;0;0;0;0;0;0;0;0;0;0;0;0;0;0;0;0;0;0;0;0;0;0;0]
      mask Display: e = 0.06;c1 = [120 230 180]/255;c2 = ([120 230 180]+0)/(256+128);c3 = ([120 230 180]+128)/(256+128);patch([0 1 1 0],[0 0 1 1],c1);patch([0 1 1 1-e 1-e 0+e],[0 0 1 1-e 0+e 0+e],c2);patch([0 0 1 1-e 0+e 0+e],[0 1 1 1-e 1-e 0+e],c3);plot([0 1 1 0 0],[0 0 1 1 0]);
  wires:
  "a{1} "/1 -> Delays 1/1("p{2}")
  Delays 1/1("pd{2,1}") -> "LW{2,1}"/1("ad{2,1}")
  "LW{2,1}"/1("lz{2,1}") -> netsum/1
  "b{2}"/1 -> netsum/2
  netsum/1 -> tansig/1
  tansig/1 -> "a{2}"/1

== system SimParking/NARX Neural Network/Layer 3 ==
  "a{2} " : Inport  PortDimensions=50  SampleTime=1
      mask Display: e = 0.06;c1 = [120 230 180]/255;c2 = ([120 230 180]+0)/(256+128);c3 = ([120 230 180]+128)/(256+128);patch([0 1 1 0],[0 0 1 1],c1);patch([0 1 1 1-e 1-e 0+e],[0 0 1 1-e 0+e 0+e],c2);patch([0 0 1 1-e 0+e 0+e],[0 1 1 1-e 1-e 0+e],c3);plot([0 1 1 0 0],[0 0 1 1 0]);
  Delays 1 : Subsystem
      mask Display: e = 0.06;c1 = [120 150 230]/255;c2 = ([120 150 230]+0)/383;c3 = ([120 150 230]+128)/383;patch([0 1 1 0],[0 0 1 1],c1);patch([0 1 1 1-e 1-e 0+e],[0 0 1 1-e 0+e 0+e],c2);patch([0 0 1 1-e 0+e 0+e],[0 1 1 1-e 1-e 0+e],c3);plot([0 1 1 0 0],[0 0 1 1 0]);disp('0');
  "LW{3,2}" : Subsystem
      mask Display: e = 0.06;c1 = [120 150 230]/255;c2 = ([120 150 230]+0)/383;c3 = ([120 150 230]+128)/383;patch([0 1 1 0],[0 0 1 1],c1);patch([0 1 1 1-e 1-e 0+e],[0 0 1 1-e 0+e 0+e],c2);patch([0 0 1 1-e 0+e 0+e],[0 1 1 1-e 1-e 0+e],c3);plot([0 1 1 0 0],[0 0 1 1 0]);disp('W');
  "b{3}" : Constant  Value=[1.6220913645536487734943875693716108798980712890625;1.517687116963644999856342110433615744113922119140625;1.5224393381279230919034262115019373595714569091796875;1.5821891447163347610427308609359897673130035400390625;1.4885275582515216097334587175282649695873260498046875;-1.2414827753449937386420742768677882850170135498046875;-1.282608006053691074299649699241854250431060791015625;1.1181175645304879395780517370440065860748291015625;-1.1886491433688330943141409079544246196746826171875;0.9910709836883293544218531678779982030391693115234375;0.94446303769535988603678333674906753003597259521484375;-0.87386977446982516681828201399184763431549072265625;0.7860843241064612296753466580412350594997406005859375;-0.8301088781182495157651146655553020536899566650390625;0.726337738391463094700384317548014223575592041015625;-0.67618780761947283597379509956226684153079986572265625;-0.43001685060995498144365001280675642192363739013671875;0.329696286813421668426826727227307856082916259765625;-0.5291423598726121557689339169883169233798980712890625;-0.44541869950729473526251922521623782813549041748046875;0.287782794581054712779177862103097140789031982421875;0.31142523121519982698401918241870589554309844970703125;-0.273483742530144346982723391192848794162273406982421875;-0.09247434042233505790964187553981901146471500396728515625;-0.0749021817889723440231364293140359222888946533203125;-0.22600388388040626441721769879222847521305084228515625;-0.07424522077722338353478193084811209701001644134521484375;0.1729478341907363103668870962792425416409969329833984375;-0.32447991011999255395181762651191093027591705322265625;0.358093519436674612155258046186645515263080596923828125;-0.28400698590420414557655703902128152549266815185546875;-0.5525671288581743834100734602543525397777557373046875;-0.1979914495481337743942873430569306947290897369384765625;-0.55039088869798291625556885264813899993896484375;-0.409757404362572075218196232526679523289203643798828125;0.4581729973095203245492257337900809943675994873046875;-0.75818872061455289124154433011426590383052825927734375;-0.8560225179111420334976401136373169720172882080078125;-0.87073289883854843029808989740558899939060211181640625;0.95601484398046243651236864025122486054897308349609375;1.088604076703236334111579708405770361423492431640625;-1.0309830403020179279138801575754769146442413330078125;-1.1579755775807567541590969995013438165187835693359375;-1.3865566977189425212912965434952639043331146240234375;-1.29015268005501493320252848207019269466400146484375;-1.331033754807700919542412520968355238437652587890625;1.5082814902466612494436049018986523151397705078125;1.610865681015226424932507143239490687847137451171875;1.6017937116494553873025097345816902816295623779296875;-1.6529061629942265465587070139008574187755584716796875]
      mask Display: e = 0.06;c1 = [120 150 230]/255;c2 = ([120 150 230]+0)/383;c3 = ([120 150 230]+128)/383;patch([0 1 1 0],[0 0 1 1],c1);patch([0 1 1 1-e 1-e 0+e],[0 0 1 1-e 0+e 0+e],c2);patch([0 0 1 1-e 0+e 0+e],[0 1 1 1-e 1-e 0+e],c3);plot([0 1 1 0 0],[0 0 1 1 0]);disp('b');
  netsum : Sum  Inputs=2  SaturateOnIntegerOverflow=on  InputSameDT=on  OutDataTypeStr=Inherit: Same as first input
      mask Display: e = 0.06;c1 = [120 150 230]/255;c2 = ([120 150 230]+0)/383;c3 = ([120 150 230]+128)/383;patch([0 1 1 0],[0 0 1 1],c1);patch([0 1 1 1-e 1-e 0+e],[0 0 1 1-e 0+e 0+e],c2);patch([0 0 1 1-e 0+e 0+e],[0 1 1 1-e 1-e 0+e],c3);plot([0 1 1 0 0],[0 0 1 1 0]);disp('+');
  tansig : neural/Transfer Functions/tansig
  "a{3}" : Outport  InitialOutput=[0;0;0;0;0;0;0;0;0;0;0;0;0;0;0;0;0;0;0;0;0;0;0;0;0;0;0;0;0;0;0;0;0;0;0;0;0;0;0;0;0;0;0;0;0;0;0;0;0;0]
      mask Display: e = 0.06;c1 = [120 230 180]/255;c2 = ([120 230 180]+0)/(256+128);c3 = ([120 230 180]+128)/(256+128);patch([0 1 1 0],[0 0 1 1],c1);patch([0 1 1 1-e 1-e 0+e],[0 0 1 1-e 0+e 0+e],c2);patch([0 0 1 1-e 0+e 0+e],[0 1 1 1-e 1-e 0+e],c3);plot([0 1 1 0 0],[0 0 1 1 0]);
  wires:
  "a{2} "/1 -> Delays 1/1("p{3}")
  Delays 1/1("pd{3,2}") -> "LW{3,2}"/1("ad{3,2}")
  "LW{3,2}"/1("lz{3,2}") -> netsum/1
  "b{3}"/1 -> netsum/2
  netsum/1 -> tansig/1
  tansig/1 -> "a{3}"/1
